simulink model "Coursework_375462_model"  (R2024b)
settings: Solver=VariableStepAuto  StartTime=0.0  StopTime=10  MaxStep=1e-4  RelTol=1e-3
undefined symbols (not defined in the file or in its folder): A_lin, B_lin, K, K_lqr, x0
settings Model: Creator=86156  LastModifiedBy=86156

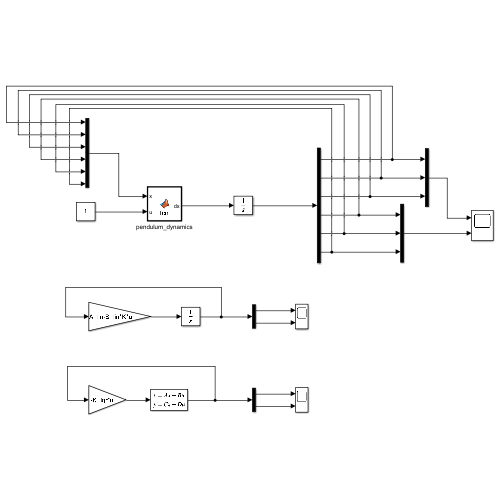
[thumbnail: Simulink's stored preview of the top-level diagram]
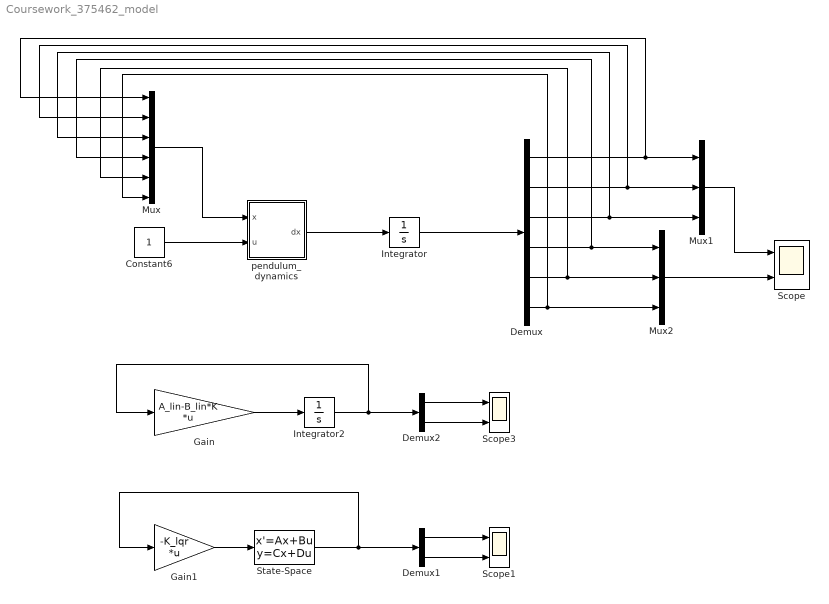
== system Coursework_375462_model ==
  Constant6 : Constant
  Demux : Demux  Outputs=6
  Demux1 : Demux  Outputs=2
  Demux2 : Demux  Outputs=2
  Gain : Gain  Gain=A_lin-B_lin*K  Multiplication=Matrix(K*u)
  Gain1 : Gain  Gain=-K_lqr  Multiplication=Matrix(K*u)
  Integrator : Integrator  InitialCondition=x0
  Integrator2 : Integrator  InitialCondition=x0
  Mux : Mux  Inputs=6
  Mux1 : Mux  Inputs=3
  Mux2 : Mux  Inputs=3
  Scope : Scope  NumInputPorts=2
  Scope1 : Scope  NumInputPorts=2
  Scope3 : Scope  NumInputPorts=2
  State-Space : StateSpace  A=A_lin  B=B_lin  C=eye(6)  D=[0; 0; 0; 0; 0; 0;]  InitialCondition=x0
  pendulum_dynamics : MATLAB Function  TreatAsAtomicUnit=on
  wires:
  Constant6/1 -> pendulum_dynamics/2(u)
  pendulum_dynamics/1(dx) -> Integrator/1
  Mux/1 -> pendulum_dynamics/1(x)
  Integrator/1 -> Demux/1
  Demux/1 -> Mux1/1, Mux/1
  Demux/2 -> Mux1/2, Mux/2
  Demux/3 -> Mux1/3, Mux/3
  Demux/4 -> Mux2/1, Mux/4
  Demux/5 -> Mux2/2, Mux/5
  Demux/6 -> Mux2/3, Mux/6
  Gain/1 -> Integrator2/1
  Integrator2/1 -> Gain/1, Demux2/1
  State-Space/1 -> Demux1/1, Gain1/1
  Gain1/1 -> State-Space/1
  Demux1/1 -> Scope1/1
  Demux1/2 -> Scope1/2
  Demux2/2 -> Scope3/2
  Demux2/1 -> Scope3/1
  Mux1/1 -> Scope/1
  Mux2/1 -> Scope/2

== matlab function Coursework_375462_model/pendulum_dynamics ==
  data: x input; dx output; u input
function dx = fcn(x, u)
    dx = f_x(x, u);
end
